simulink model "Landing_Check_1_Harness2"  (R2023a)
settings: Solver=FixedStepAuto  StartTime=0.0  StopTime=0.  FixedStep=1.  RelTol=1e-3
settings Model: Creator=horty  LastModifiedBy=horty
settings DataIOCC: SignalLogging=off  DSMLogging=off  SaveTime=off  ReturnWorkspaceOutputs=off

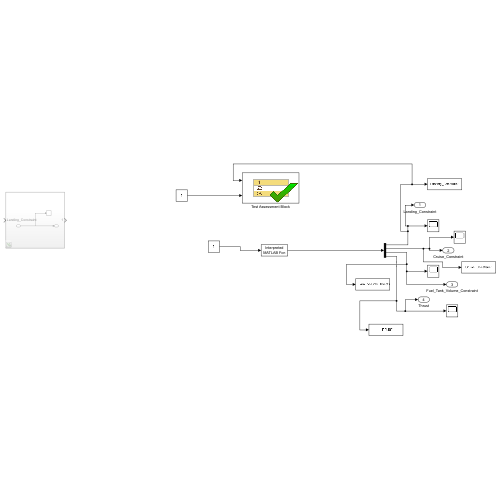
[thumbnail: Simulink's stored preview of the top-level diagram]
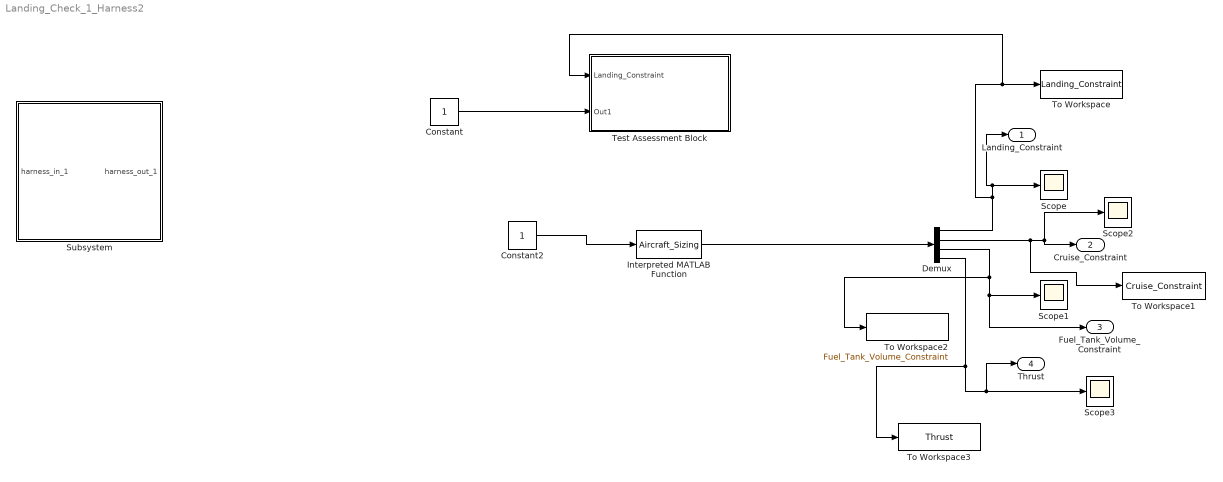
== system Landing_Check_1_Harness2 ==
  Constant : Constant
  Constant2 : Constant
  Demux : Demux
  Interpreted MATLAB Function : MATLABFcn  MATLABFcn=Aircraft_Sizing  OutputSignalType=real
  Scope{,1..3} (4 alike) : Scope
  Subsystem : Subsystem  Tag=__SL_testing_harness_stub_
  Test Assessment Block : Test Sequence  Tag=__SLT_ASMT__  TreatAsAtomicUnit=on
  To Workspace : ToWorkspace  VariableName=Landing_Constraint  SampleTime=-1
  To Workspace1 : ToWorkspace  VariableName=Cruise_Constraint  SampleTime=-1
  To Workspace2 : ToWorkspace  VariableName=Fuel_Tank_Volume_Constraint  SampleTime=-1
  To Workspace3 : ToWorkspace  VariableName=Thrust  SampleTime=-1
  Landing_Constraint : Outport
  Cruise_Constraint : Outport  Port=2
  Fuel_Tank_Volume_Constraint : Outport  Port=3
  Thrust : Outport  Port=4
  wires:
  Demux/1 -> Test Assessment Block/1(Landing_Constraint), To Workspace/1, Scope/1, Landing_Constraint/1
  Constant/1 -> Test Assessment Block/2(Out1)
  Interpreted MATLAB Function/1 -> Demux/1
  Constant2/1 -> Interpreted MATLAB Function/1
  Demux/2 -> To Workspace1/1, Cruise_Constraint/1, Scope2/1
  Demux/4 -> To Workspace3/1, Thrust/1, Scope3/1
  Demux/3 -> To Workspace2/1, Fuel_Tank_Volume_Constraint/1, Scope1/1

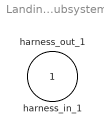
== system Landing_Check_1_Harness2/Subsystem ==
  harness_in_1 : Inport
  harness_out_1 : Outport

== stateflow chart Landing_Check_1_Harness2/Test Assessment Block ==
  state Assessments
    state step_1_1
      verify(Landing_Constraint<-400)
    state Else
    (default) -> (junction 22)
    Assessments -> (junction 22)
    (junction 22) -> (junction 23) [order 1] : [(Out1==1)
        | ]
    (junction 23) -> step_1_1 [order 1] : [~in(Assessments.step_1_1)]
    (junction 22) -> (junction 31) [order 2]
    (junction 23) -> (junction 26) [order 2]
    (junction 31) -> (junction 32)
    (junction 32) -> Else [order 1] : [~in(Assessments.Else)]
    (junction 32) -> (junction 35) [order 2]
  (default) -> Assessments
  data: Landing_Constraint input double size=[1]; Out1 input double size=[1]
